simulink model "batida_morta"  (R2022b)
settings: Solver=VariableStepAuto  StartTime=0.0  StopTime=10.0  RelTol=1e-3
values from neighbouring files (symbols this model uses):
  den_dead = [1,-p]    [lab9e10.m]
  R = 1.18    [lab9e10.m]
  T0 = 0.01    [lab9e10.m]
undefined symbols (not defined in the file or in its folder): d, den, num, num_dead, t1
settings Model: Creator=coveiro  LastModifiedBy=coveiro

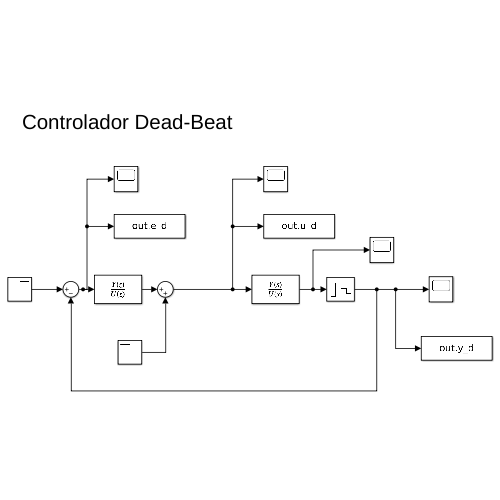
[thumbnail: Simulink's stored preview of the top-level diagram]
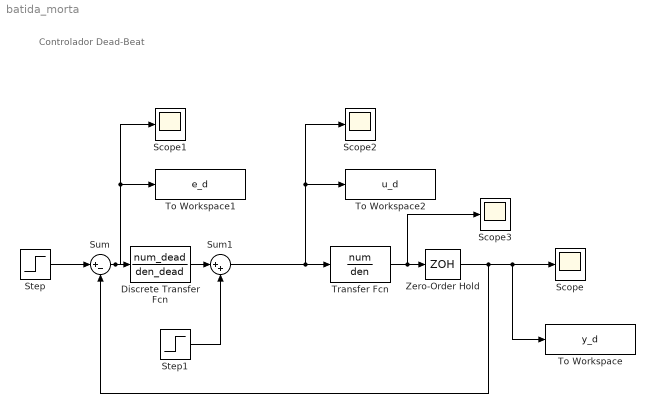
== system batida_morta ==
  note: Controlador Dead-Beat
  Discrete Transfer Fcn : DiscreteTransferFcn  Numerator=num_dead  Denominator=den_dead  SampleTime=T0
  Scope{,1..3} (4 alike) : Scope
  Step : Step  Time=0  After=R  SampleTime=0
  Step1 : Step  Time=t1  After=d  SampleTime=0
  Sum : Sum  Inputs=|+-
  Sum1 : Sum  Inputs=|++
  To Workspace : ToWorkspace  VariableName=y_d  SaveFormat=Timeseries  SampleTime=-1
  To Workspace1 : ToWorkspace  VariableName=e_d  SaveFormat=Timeseries  SampleTime=-1
  To Workspace2 : ToWorkspace  VariableName=u_d  SaveFormat=Timeseries  SampleTime=-1
  Transfer Fcn : TransferFcn  Numerator=num  Denominator=den
  Zero-Order Hold : ZeroOrderHold  SampleTime=T0
  wires:
  Transfer Fcn/1 -> Scope3/1, Zero-Order Hold/1
  Step1/1 -> Sum1/2
  Sum1/1 -> To Workspace2/1, Scope2/1, Transfer Fcn/1
  Zero-Order Hold/1 -> Sum/2, To Workspace/1, Scope/1
  Step/1 -> Sum/1
  Sum/1 -> To Workspace1/1, Scope1/1, Discrete Transfer Fcn/1
  Discrete Transfer Fcn/1 -> Sum1/1
